simulink model "IM_CurrentControllerDesign_vdqsat"  (R2024b)
settings: Solver=VariableStepAuto  StartTime=0.0  StopTime=1e-3  RelTol=1e-3
undefined symbols (not defined in the file): ctrl, en_d, en_q, im, iSd_step, iSq_step, Ts
libraries: simulink x2, cstblocks x2
settings Model: Creator=overflow  LastModifiedBy=matth

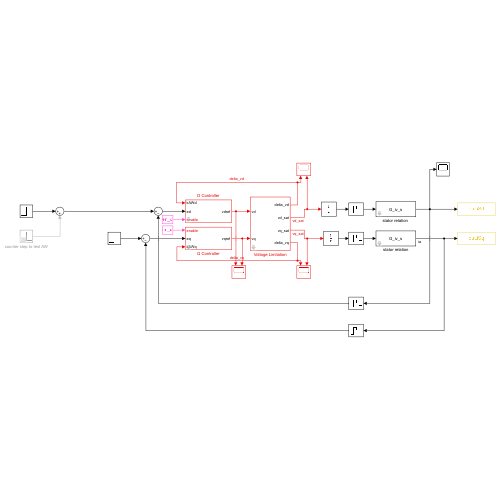
[thumbnail: Simulink's stored preview of the top-level diagram]
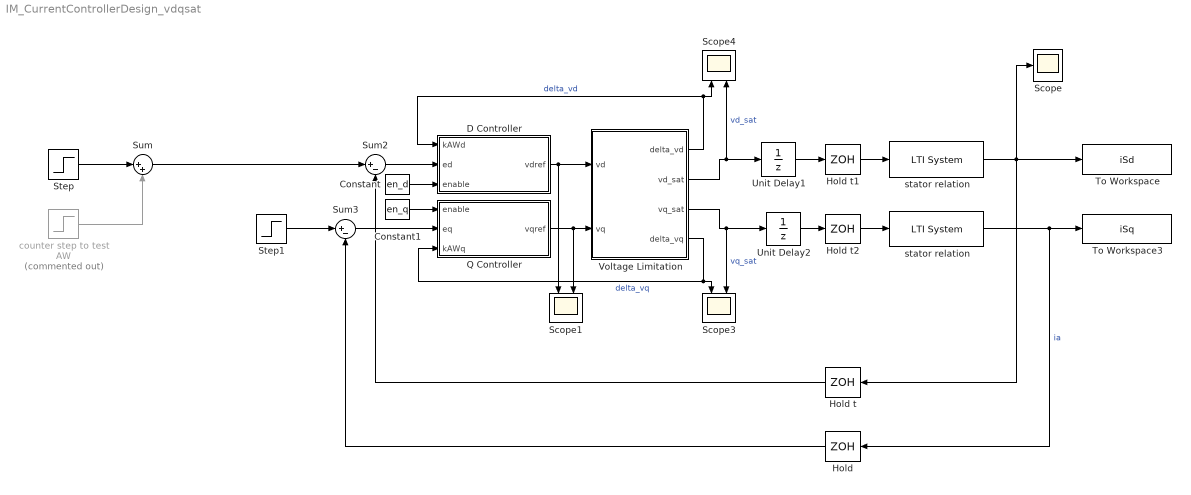
== system IM_CurrentControllerDesign_vdqsat ==
  " Hold" : ZeroOrderHold  SampleTime=Ts
  " Hold t" : ZeroOrderHold  SampleTime=Ts
  " Hold t1" : ZeroOrderHold  SampleTime=Ts
  " Hold t2" : ZeroOrderHold  SampleTime=Ts
  Constant : Constant  Value=en_d
  Constant1 : Constant  Value=en_q
  D Controller : Subsystem  mask{Ts=ctrl.Ts, ctrl=ctrl.i}
      mask prompts: Ts "Sampling Time"; ctrl "Controller Struct"
  Q Controller : Subsystem  mask{Ts=ctrl.Ts, ctrl=ctrl.i}
      mask prompts: Ts "Sampling Time"; ctrl "Controller Struct"
  Scope : Scope
  Scope1 : Scope  NumInputPorts=2
  Scope3 : Scope  NumInputPorts=2
  Scope4 : Scope  NumInputPorts=2
  Step : Step  Time=0  After=iSd_step  SampleTime=0
  Step1 : Step  Time=0  After=iSq_step  SampleTime=0
  Sum : Sum  Inputs=|++
  Sum2 : Sum  Inputs=|+-
  Sum3 : Sum  Inputs=|+-
  To Workspace : ToWorkspace  VariableName=iSd  SaveFormat=Timeseries  SampleTime=-1
  To Workspace3 : ToWorkspace  VariableName=iSq  SaveFormat=Timeseries  SampleTime=-1
  Unit Delay1 : UnitDelay  SampleTime=Ts  HasFrameUpgradeWarning=on
  Unit Delay2 : UnitDelay  SampleTime=Ts  HasFrameUpgradeWarning=on
  Voltage Limitation : Subsystem  mask{Vmax=im.vSmax}
      mask prompts: Vmax "Max Voltage"
  counter step to test AW : Step  Commented=on  Time=10e-3  After=-55  SampleTime=0
  stator relation : cstblocks/LTI System  sys=G_iv_s  IC=[0]  PadeOrder=0
  "stator relation " : cstblocks/LTI System  sys=G_iv_s  IC=[0]  PadeOrder=0
  wires:
  Sum2/1 -> D Controller/2(ed)
  Sum3/1 -> Q Controller/2(eq)
  " Hold t"/1 -> Sum2/2
  " Hold t1"/1 -> "stator relation "/1
  " Hold t2"/1 -> stator relation/1
  " Hold"/1 -> Sum3/2
  "stator relation "/1 -> " Hold t"/1, Scope/1, To Workspace/1
  stator relation/1 -> To Workspace3/1, " Hold"/1  "ia"
  Unit Delay2/1 -> " Hold t2"/1
  Unit Delay1/1 -> " Hold t1"/1
  Voltage Limitation/3(vq_sat) -> Unit Delay2/1, Scope3/2  "vq_sat"
  Voltage Limitation/2(vd_sat) -> Scope4/2, Unit Delay1/1  "vd_sat"
  Q Controller/1(vqref) -> Scope1/2, Voltage Limitation/2("vq ")
  D Controller/1(vdref) -> Scope1/1, Voltage Limitation/1(vd)
  Constant/1 -> D Controller/3(enable)
  Voltage Limitation/1(delta_vd) -> Scope4/1, D Controller/1(kAWd)  "delta_vd"
  Voltage Limitation/4(delta_vq) -> Scope3/1, Q Controller/3(kAWq)  "delta_vq"
  Step1/1 -> Sum3/1
  Sum/1 -> Sum2/1
  Constant1/1 -> Q Controller/1(enable)
  Step/1 -> Sum/1
  counter step to test AW/1 -> Sum/2

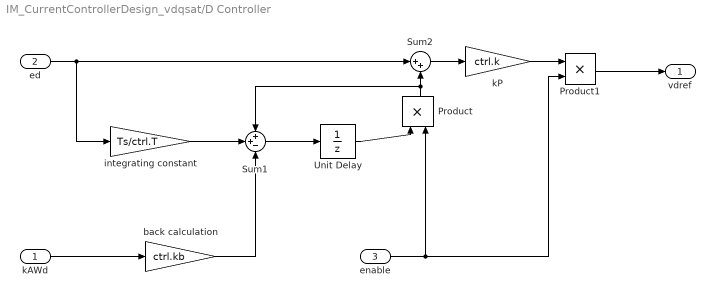
== system IM_CurrentControllerDesign_vdqsat/D Controller ==
  kAWd : Inport
  ed : Inport  Port=2
  enable : Inport  Port=3
  Product : Product
  Product1 : Product
  Sum1 : Sum  Inputs=++-
  Sum2 : Sum  Inputs=|++
  Unit Delay : UnitDelay  SampleTime=-1  HasFrameUpgradeWarning=on
  back calculation : Gain  Gain=ctrl.kb
  integrating constant : Gain  Gain=Ts/ctrl.T
  kP : Gain  Gain=ctrl.k
  vdref : Outport
  wires:
  ed/1 -> integrating constant/1, Sum2/1
  Sum2/1 -> kP/1
  kAWd/1 -> back calculation/1
  Sum1/1 -> Unit Delay/1
  Unit Delay/1 -> Product/1
  Product/1 -> Sum1/1, Sum2/2
  kP/1 -> Product1/1
  Product1/1 -> vdref/1
  enable/1 -> Product1/2, Product/2
  integrating constant/1 -> Sum1/2
  back calculation/1 -> Sum1/3

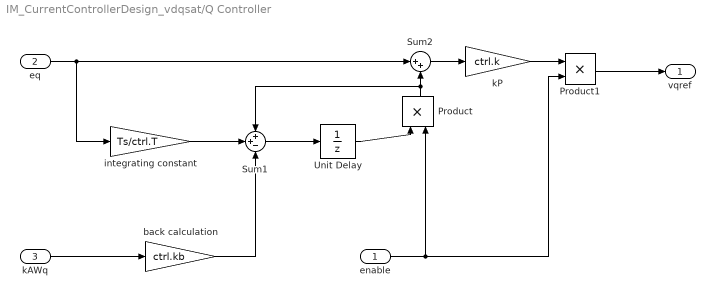
== system IM_CurrentControllerDesign_vdqsat/Q Controller ==
  enable : Inport
  eq : Inport  Port=2
  kAWq : Inport  Port=3
  Product : Product
  Product1 : Product
  Sum1 : Sum  Inputs=++-
  Sum2 : Sum  Inputs=|++
  Unit Delay : UnitDelay  SampleTime=-1  HasFrameUpgradeWarning=on
  back calculation : Gain  Gain=ctrl.kb
  integrating constant : Gain  Gain=Ts/ctrl.T
  kP : Gain  Gain=ctrl.k
  vqref : Outport
  wires:
  eq/1 -> integrating constant/1, Sum2/1
  Sum2/1 -> kP/1
  kAWq/1 -> back calculation/1
  Sum1/1 -> Unit Delay/1
  Unit Delay/1 -> Product/1
  Product/1 -> Sum1/1, Sum2/2
  kP/1 -> Product1/1
  Product1/1 -> vqref/1
  enable/1 -> Product1/2, Product/2
  integrating constant/1 -> Sum1/2
  back calculation/1 -> Sum1/3

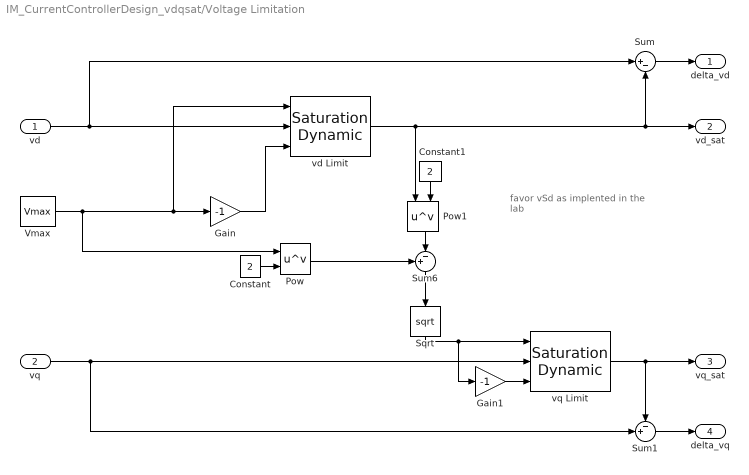
== system IM_CurrentControllerDesign_vdqsat/Voltage Limitation ==
  note: favor vSd as implented in the lab
  vd : Inport
  "vq " : Inport  Port=2
  Constant : Constant  Value=2
  Constant1 : Constant  Value=2
  Gain : Gain  Gain=-1
  Gain1 : Gain  Gain=-1
  Pow : Math  Operator=pow  RndMeth=Zero
  Pow1 : Math  Operator=pow  RndMeth=Zero
  Sqrt : Sqrt
  Sum : Sum  Inputs=|+-
  Sum1 : Sum  Inputs=-+|
  Sum6 : Sum  Inputs=+-|
  Vmax : Constant  Value=Vmax
  vd Limit : simulink/Discontinuities/Saturation Dynamic  OutMin=[]  OutMax=[]  OutDataTypeStr=Inherit: Same as second input  OutDataType=fixdt(1, 16)  OutScaling=2^-10  DoSatur=off
  vq Limit : simulink/Discontinuities/Saturation Dynamic  OutMin=[]  OutMax=[]  OutDataTypeStr=Inherit: Same as second input  OutDataType=fixdt(1, 16)  OutScaling=2^-10  DoSatur=off
  delta_vd : Outport  VectorParamsAs1DForOutWhenUnconnected=off
  vd_sat : Outport  Port=2  VectorParamsAs1DForOutWhenUnconnected=off
  vq_sat : Outport  Port=3  VectorParamsAs1DForOutWhenUnconnected=off
  delta_vq : Outport  Port=4  VectorParamsAs1DForOutWhenUnconnected=off
  wires:
  Gain/1 -> vd Limit/3
  vd Limit/1 -> Sum/2, vd_sat/1, Pow1/1
  Sqrt/1 -> Gain1/1, vq Limit/1
  vq Limit/1 -> Sum1/1, vq_sat/1
  Pow/1 -> Sum6/1
  vd/1 -> Sum/1, vd Limit/2
  Sum6/1 -> Sqrt/1
  "vq "/1 -> vq Limit/2, Sum1/2
  Pow1/1 -> Sum6/2
  Vmax/1 -> Pow/1, Gain/1, vd Limit/1
  Gain1/1 -> vq Limit/3
  Sum/1 -> delta_vd/1
  Sum1/1 -> delta_vq/1
  Constant/1 -> Pow/2
  Constant1/1 -> Pow1/2
